simulink model "s_3d_crane_payload_pos_cntrl"  (Simulink 6.6)
settings: Solver=FixedStepDiscrete  StartTime=0.0  StopTime=10  FixedStep=0.001  RelTol=1e-3
values from neighbouring files (symbols this model uses):
  eff_g_y = 1    [config_3d_crane.m]
  eff_m_y = 0.81    [config_3d_crane.m]
  g = 9.81    [config_3d_crane.m]
  IMAX_AMP = 7    [setup_3d_crane.m]
  J_phi = Jm_y + J_y_reel    [config_3d_crane.m]
  Kg_y = Kg_y_i*Kg_y_e    (= 28)    [config_3d_crane.m]
  ki = w0^2*p0*(mp*r_y_reel^2+J_phi)/eff_g_y/Kg_y/eff_m_y/Kt_y/r_y_reel    [d_payload_piv_controller.m]
  kp = w0*(2*zeta*p0*J_phi+w0*mp*r_y_reel^2+w0*J_phi+2*zeta*p0*mp*r_y_reel^2)/eff_g_y/Kg_y/eff_m_y/Kt_y/r_y_reel    [d_payload_piv_controller.m]
  Kt_y = 0.0261    [config_3d_crane.m]
  kv = (p0*J_phi+2*zeta*w0*mp*r_y_reel^2+2*zeta*w0*J_phi+p0*mp*r_y_reel^2)/eff_g_y/Kg_y/eff_m_y/Kt_y/r_y_reel    [d_payload_piv_controller.m]
  mp = 0.147    [config_3d_crane.m]
  r_y_reel = 1.0 / 2 * K_IN2M    [config_3d_crane.m]
  wf_z = 2 * pi * 50    (= 314.159265359)    [setup_3d_crane.m]
undefined symbols (not defined in the file or in its folder): DiscIntNeverNeededParam, qc_get_step_size
libraries: quarc_library x2, simulink x1
settings Model: Creator=MLevis  LastModifiedBy=MLevis  ExtModeTrigDuration=10000
settings SolverCC: PositivePriorityOrder=on
settings RTWCC: SystemTargetFile=quarc_windows.tlc  TemplateMakefile=quarc_default_tmf  Description=QuaRC Win32 Target  ProcessScript=quarc_windows_make_rtw_hook
settings STFCustomTargetCC: TargetFcnLib=ansi_tfl_tmw.mat  TargetPreCompLibLocation=C:\DOCUME~1\ALLUSE~1\APPLIC~1\QuaRC\lib\2007a\windows\release  GenFloatMathFcnCalls=ANSI_C  SystemTargetFile=quarc_windows.tlc
settings GRTTargetCC: TargetPreCompLibLocation=C:\DOCUME~1\ALLUSE~1\APPLIC~1\QuaRC\lib\2007a\windows\release  MatFileLogging=off  ExtMode=on  ExtModeMexFile=quarc_comm

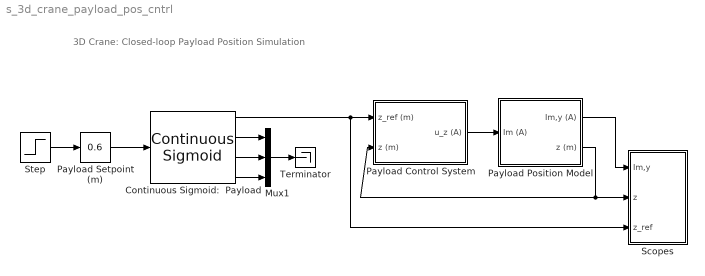
== system s_3d_crane_payload_pos_cntrl ==
  note: 3D Crane: Closed-loop Payload Position Simulation
  Continuous Sigmoid:  Payload : quarc_library/Sources/Sigmoids/Continuous Sigmoid  params_source=Internal (dialog parameters)  max_velocity=0.25  max_acceleration=0.25  initial_position=0  initial_velocity=0  hold_off=0.5  input_sample_time=-1  output_sample_time=qc_get_step_size
  Mux1 : Mux  Inputs=3
  Payload Control System : Subsystem
  Payload Position Model : Subsystem
  Payload Setpoint (m) : simulink/Math Operations/Slider Gain  SystemSampleTime=-1  low=-0.5  gain=0.6  high=0.6
  Scopes : Subsystem
  Step : Step  SampleTime=0
  Terminator : Terminator
  wires:
  Payload Control System/1(u_z (A)) -> Payload Position Model/1(Im (A))
  Continuous Sigmoid:  Payload/1 -> Payload Control System/1(z_ref (m)), Scopes/3(z_ref)
  Payload Setpoint (m)/1 -> Continuous Sigmoid:  Payload/1
  Step/1 -> Payload Setpoint (m)/1
  Payload Position Model/2(z (m)) -> Payload Control System/2(z (m)), Scopes/2(z)
  Mux1/1 -> Terminator/1
  Continuous Sigmoid:  Payload/2 -> Mux1/1
  Continuous Sigmoid:  Payload/3 -> Mux1/2
  Continuous Sigmoid:  Payload/4 -> Mux1/3
  Payload Position Model/1(Im,y (A)) -> Scopes/1(Im,y)

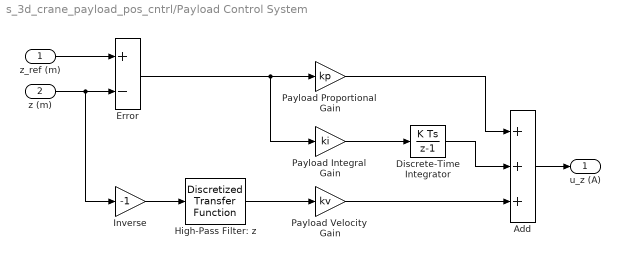
== system s_3d_crane_payload_pos_cntrl/Payload Control System ==
  z_ref (m) : Inport
  z (m) : Inport  Port=2
  Add : Sum  Inputs=+++  OutScaling=2^-10
  Discrete-Time Integrator : DiscreteIntegrator  SampleTime=qc_get_step_size  ICPrevOutput=DiscIntNeverNeededParam  ICPrevScaledInput=DiscIntNeverNeededParam
  Error : Sum  Inputs=+-  OutScaling=2^-10
  High-Pass Filter: z : quarc_library/Discrete/Discretized Transfer Function  SystemSampleTime=-1  num=[wf_z 0]  den=[1 wf_z]  method=tustin  Ts=qc_get_step_size
  Inverse : Gain  Gain=-1
  Payload Integral  Gain : Gain  Gain=ki
  Payload Proportional  Gain : Gain  Gain=kp
  Payload Velocity  Gain : Gain  Gain=kv
  u_z (A) : Outport
  wires:
  Payload Velocity  Gain/1 -> Add/3
  Error/1 -> Payload Integral  Gain/1, Payload Proportional  Gain/1
  Discrete-Time Integrator/1 -> Add/2
  Payload Proportional  Gain/1 -> Add/1
  Add/1 -> u_z (A)/1
  Payload Integral  Gain/1 -> Discrete-Time Integrator/1
  z_ref (m)/1 -> Error/1
  z (m)/1 -> Error/2, Inverse/1
  High-Pass Filter: z/1 -> Payload Velocity  Gain/1
  Inverse/1 -> High-Pass Filter: z/1

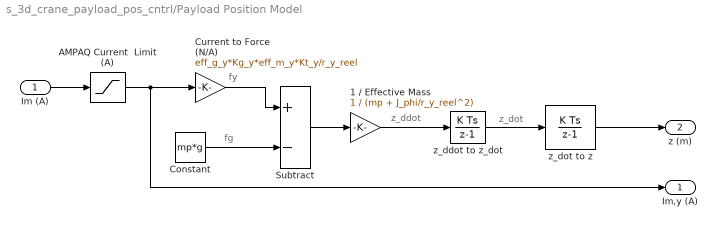
== system s_3d_crane_payload_pos_cntrl/Payload Position Model ==
  note: z_ddot
  note: z_dot
  note: fy
  note: fg
  Im (A) : Inport
  1 / Effective Mass : Gain  Gain=1 / (mp + J_phi/r_y_reel^2)
  AMPAQ Current  Limit (A) : Saturate  UpperLimit=IMAX_AMP  LowerLimit=-IMAX_AMP
  Constant : Constant  Value=mp*g
  Current to Force (N/A) : Gain  Gain=eff_g_y*Kg_y*eff_m_y*Kt_y/r_y_reel
  Subtract : Sum  Inputs=+-  OutScaling=2^-10
  z_ddot to z_dot : DiscreteIntegrator  SampleTime=qc_get_step_size  ICPrevOutput=DiscIntNeverNeededParam  ICPrevScaledInput=DiscIntNeverNeededParam
  z_dot to z : DiscreteIntegrator  SampleTime=qc_get_step_size  LimitOutput=on  UpperSaturationLimit=32*0.0254  LowerSaturationLimit=0  ICPrevOutput=DiscIntNeverNeededParam  ICPrevScaledInput=DiscIntNeverNeededParam
  Im,y (A) : Outport
  z (m) : Outport  Port=2
  wires:
  Im (A)/1 -> AMPAQ Current  Limit (A)/1
  Constant/1 -> Subtract/2
  Current to Force (N/A)/1 -> Subtract/1
  Subtract/1 -> 1 / Effective Mass/1
  1 / Effective Mass/1 -> z_ddot to z_dot/1
  z_ddot to z_dot/1 -> z_dot to z/1
  z_dot to z/1 -> z (m)/1
  AMPAQ Current  Limit (A)/1 -> Current to Force (N/A)/1, Im,y (A)/1

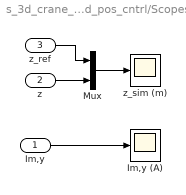
== system s_3d_crane_payload_pos_cntrl/Scopes ==
  Im,y : Inport
  z : Inport  Port=2
  z_ref : Inport  Port=3
  Im,y (A) : Scope
      settings: TimeRange=10  YMin=-0.5  YMax=2.5  SaveName=ScopeData2
  Mux : Mux  Inputs=2
  z_sim (m) : Scope
      settings: TimeRange=10  YMin=0  YMax=0.7000000000000001
  wires:
  Mux/1 -> z_sim (m)/1
  z_ref/1 -> Mux/1
  z/1 -> Mux/2
  Im,y/1 -> Im,y (A)/1
